simulink model "DiscreteModel"  (R2019b)
settings: Solver=ode4  StartTime=0.0  StopTime=SimTime  FixedStep=0.01  RelTol=1e-3  EnableMultiTasking=on
values from neighbouring files (symbols this model uses):
  A = (1+r/m)^(m*n)    (= 1.12699211369)    [Script.m]
  B = 0    [Script.m]
  C = 1    [Script.m]
  D = 0    [Script.m]
  IC = 10    [Script.m]
  Step = 1/m    (= 0.25)    [Script.m]
settings Model: Creator=falcon  LastModifiedBy=Illia Bannitsyn
settings DataIOCC: LimitDataPoints=on

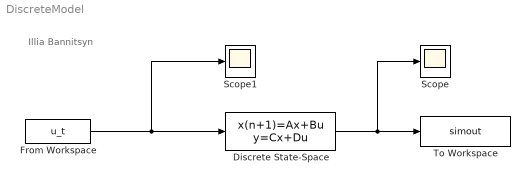
== system DiscreteModel ==
  note: Illia Bannitsyn
  Discrete State-Space : DiscreteStateSpace  A=A  B=B  C=C  D=D  InitialCondition=IC  SampleTime=-1
  From Workspace : FromWorkspace  VariableName=u_t  SampleTime=Step
  Scope : Scope
  Scope1 : Scope
  To Workspace : ToWorkspace  VariableName=simout  SaveFormat=Timeseries  SampleTime=-1
      settings: Save2DSignal=2-D array (concatenate along first dimension)
  wires:
  From Workspace/1 -> Scope1/1, Discrete State-Space/1
  Discrete State-Space/1 -> Scope/1, To Workspace/1
